simulink model "modulador_de_torque"  (R2018a)
settings: Solver=VariableStepAuto  StartTime=0.0  StopTime=10.0  RelTol=1e-3
values from neighbouring files (symbols this model uses):
  b_eq = b_m + b_l/r^2    (= 1.5e-05)    [proyecto_global_integrador.m]
  L_d = 6.6e-3    (= 0.0066)    [proyecto_global_integrador.m]
  L_q = 5.8e-3    (= 0.0058)    [proyecto_global_integrador.m]
  lambda_m = 0.01546    [proyecto_global_integrador.m]
  P_p = 3    [proyecto_global_integrador.m]
  R_s = 1.02    [polos_choreo_no_se_puede_robar_mas_con_esto.m]    (also in proyecto_global_integrador.m)
  Rp_0 = 4    [proyecto_global_integrador.m]
  Rp_d = 33    [proyecto_global_integrador.m]
  Rp_q = 29    [proyecto_global_integrador.m]
settings Model: Creator=gabrielq  LastModifiedBy=gabrielq

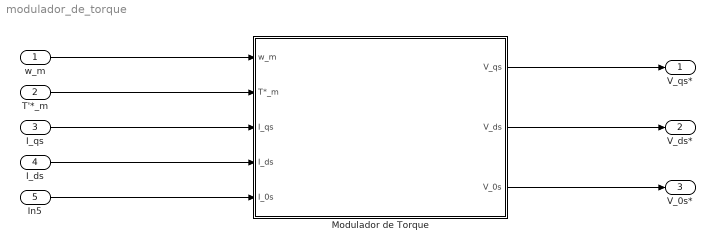
== system modulador_de_torque ==
  w_m : Inport
  T'*_m : Inport  Port=2
  I_qs : Inport  Port=3
  I_ds : Inport  Port=4
  In5 : Inport  Port=5
  Modulador de Torque : Subsystem
  V_qs* : Outport
  V_ds* : Outport  Port=2
  V_0s* : Outport  Port=3
  wires:
  w_m/1 -> Modulador de Torque/1(w_m)
  T'*_m/1 -> Modulador de Torque/2(T*_m)
  I_qs/1 -> Modulador de Torque/3(I_qs)
  I_ds/1 -> Modulador de Torque/4(I_ds)
  In5/1 -> Modulador de Torque/5(I_0s)
  Modulador de Torque/1(V_qs) -> V_qs*/1
  Modulador de Torque/2(V_ds) -> V_ds*/1
  Modulador de Torque/3(V_0s) -> V_0s*/1

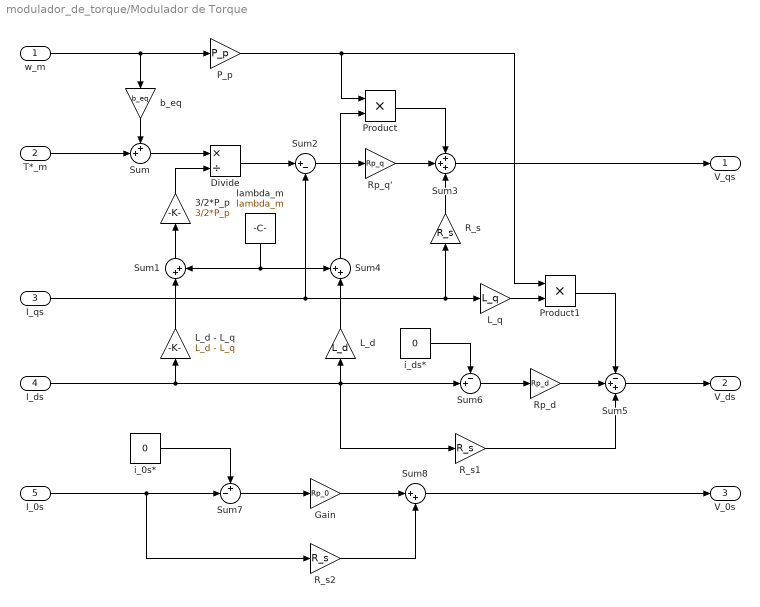
== system modulador_de_torque/Modulador de Torque ==
  w_m : Inport
  T*_m : Inport  Port=2
  I_qs : Inport  Port=3
  I_ds : Inport  Port=4
  I_0s : Inport  Port=5
  " lambda_m" : Constant  Value=lambda_m
  3/2*P_p : Gain  Gain=3/2*P_p
  Divide : Product  Inputs=*/
  Gain : Gain  Gain=Rp_0
  L_d : Gain  Gain=L_d
  L_d - L_q : Gain  Gain=L_d - L_q
  L_q : Gain  Gain=L_q
  P_p : Gain  Gain=P_p
  Product : Product
  Product1 : Product
  R_s : Gain  Gain=R_s
  R_s1 : Gain  Gain=R_s
  R_s2 : Gain  Gain=R_s
  Rp_d : Gain  Gain=Rp_d
  Rp_q' : Gain  Gain=Rp_q
  Sum : Sum  Inputs=++|
  Sum1 : Sum  Inputs=|++
  Sum2 : Sum  Inputs=|+-
  Sum3 : Sum  Inputs=+++
  Sum4 : Sum  Inputs=++|
  Sum5 : Sum  Inputs=-++
  Sum6 : Sum  Inputs=-+|
  Sum7 : Sum  Inputs=+-|
  Sum8 : Sum  Inputs=|++
  "b_eq " : Gain  Gain=b_eq
  i_0s* : Constant  Value=0
  i_ds* : Constant  Value=0
  V_qs : Outport
  V_ds : Outport  Port=2
  V_0s : Outport  Port=3
  wires:
  T*_m/1 -> Sum/2
  R_s2/1 -> Sum8/2
  Product1/1 -> Sum5/1
  i_0s*/1 -> Sum7/1
  Product/1 -> Sum3/1
  Sum/1 -> Divide/1
  L_d - L_q/1 -> Sum1/1
  R_s1/1 -> Sum5/3
  w_m/1 -> P_p/1, "b_eq "/1
  "b_eq "/1 -> Sum/1
  Rp_d/1 -> Sum5/2
  " lambda_m"/1 -> Sum4/1, Sum1/2
  L_q/1 -> Product1/2
  Sum6/1 -> Rp_d/1
  I_0s/1 -> R_s2/1, Sum7/2
  P_p/1 -> Product1/1, Product/1
  i_ds*/1 -> Sum6/1
  Gain/1 -> Sum8/1
  L_d/1 -> Sum4/2
  Sum8/1 -> V_0s/1
  Sum5/1 -> V_ds/1
  Sum2/1 -> Rp_q'/1
  Divide/1 -> Sum2/1
  Sum1/1 -> 3/2*P_p/1
  I_ds/1 -> R_s1/1, Sum6/2, L_d/1, L_d - L_q/1
  Sum4/1 -> Product/2
  Sum3/1 -> V_qs/1
  3/2*P_p/1 -> Divide/2
  Rp_q'/1 -> Sum3/2
  R_s/1 -> Sum3/3
  I_qs/1 -> Sum2/2, L_q/1, R_s/1
  Sum7/1 -> Gain/1
